simulink model "TCS_test_2"  (R2026a)
settings: Solver=ode4  StartTime=0  StopTime=5  FixedStep=0.0005
model workspace (MAT data in the model file):
  P.g = 9.81
  P.vehicleMass = 310
  P.channelMass = 155
  P.rearStaticFraction = 0.5
  P.wheelbase = 1.55
  P.cgHeight = 0.289
  P.tyreRadius = 0.25908
  P.gearRatio = 6
  P.drivetrainEfficiency = 0.95
  P.differentialSplit = 0.5
  P.motorPeakTorque = 220
  P.motorPeakPower = 80000
  P.motorMaximumRPM = 5170
  P.motorTimeConstant = 0.02
  P.wheelEquivalentInertia = 0.9
  P.rollingResistance = 0.015
  P.airDensity = 1.225
  P.dragArea = 0.8
  P.magicB = 10
  P.magicC = 1.9
  P.magicE = 0.97
  P.actualMuDry = 1.2
  P.actualMuLow = 0.48
  P.estimatedMuDry = 1.05
  P.estimatedMuLow = 0.58
  P.gripChangeTime = 1.5
  P.controllerSampleTime = 0.002
  P.plantStep = 0.0005
  P.stopTime = 5
  P.slipDenominatorGuard = 0.5
  P.slipFilterTimeConstant = 0.015
  P.slipTarget = 0.12
  P.slipActivation = 0.14
  P.slipRelease = 0.09
  P.activationPersistence = 0.02
  P.releasePersistence = 0.08
  P.recoveryTime = 0.12
  P.controlEnableSpeed = 1.5
  P.launchSlipVelocity = 0.35
  P.launchVelocityGain = 80
  P.launchTorqueCap = 85
  P.admissibleTorqueSafetyFactor = 0.95
  P.Kp = 650
  P.Ki = 900
  P.Kaw = 0.00153846153846
  P.integratorMinimum = -0.35
  P.integratorMaximum = 0.1
  P.torqueCutRate = 9000
  P.torqueRestoreRate = 500
  P.sensorResolutionRPM = 0.25
  P.faultTorque = 0
  driverProfile = [0  0; 0.2  0; 0.8  1; 2.8  1; 3  0; 3.3  0; 3.5  -0.8; 5.5  -0.8; 6  0]
  roadProfile = [0  1.2; 1.5  0.7; 2  1.2; 4  0.7; 4.5  1.2; 6  1.2]
libraries: simulink x1
Description:
  | Interactive single-wheel EV traction-control model.
  | Generated by build_TCS_test_2_simulink.m.
  | Proactive admissible torque plus reactive slip control.
settings Model: Creator=Arulm  LastModifiedBy=Arulm
settings DebuggingCC: AlgebraicLoopMsg=error  UnconnectedInputMsg=error  UnconnectedOutputMsg=error

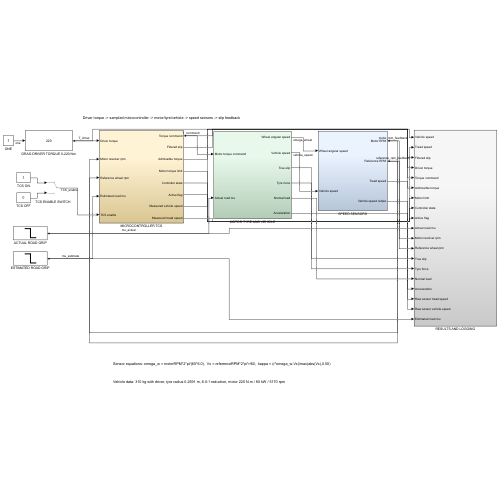
[thumbnail: Simulink's stored preview of the top-level diagram]
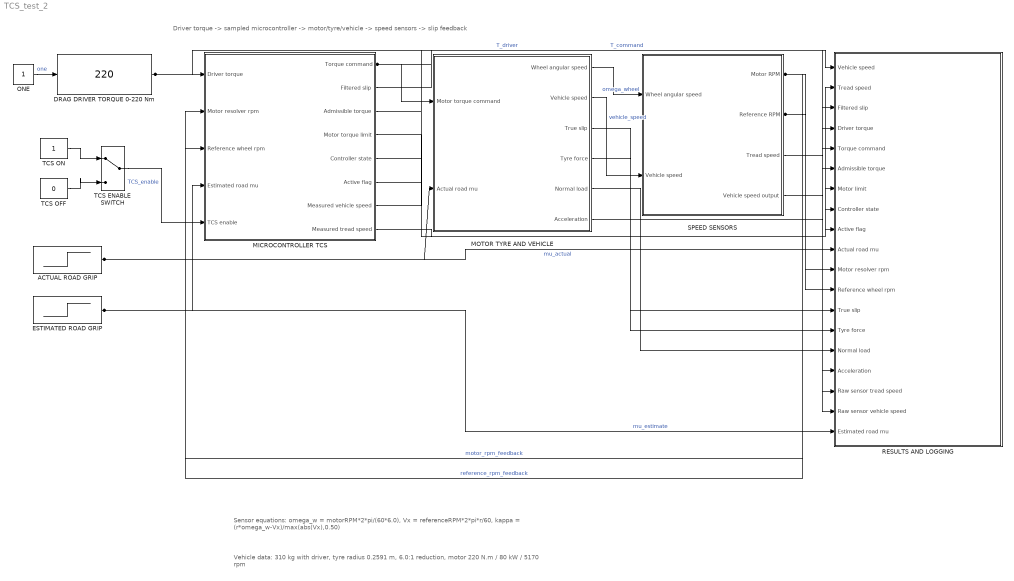
== system TCS_test_2 ==
  note: Driver torque -> sampled microcontroller -> motor/tyre/vehicle -> speed sensors -> slip feedback
  note: Sensor equations: omega_w = motorRPM*2*pi/(60*6.0), Vx = referenceRPM*2*pi*r/60, kappa = (r*omega_w-Vx)/max(abs(Vx),0.50)
  note: Vehicle data: 310 kg with driver, tyre radius 0.2591 m, 6.0:1 reduction, motor 220 N.m / 80 kW / 5170 rpm
  ACTUAL ROAD GRIP : Step  Time=1.5  InitialValue=1.2  FinalValue=0.48  SampleTime=0
  DRAG DRIVER TORQUE 0-220 Nm : simulink/Math Operations/Slider Gain  gain=220  low=0  high=220
  ESTIMATED ROAD GRIP : Step  Time=1.5  InitialValue=1.05  FinalValue=0.58  SampleTime=0
  MICROCONTROLLER TCS : Subsystem
  MOTOR TYRE AND VEHICLE : Subsystem
  ONE : Constant
  RESULTS AND LOGGING : Subsystem
  SPEED SENSORS : Subsystem
  TCS ENABLE SWITCH : ManualSwitch
  TCS OFF : Constant  Value=0  OutDataTypeStr=boolean
  TCS ON : Constant  OutDataTypeStr=boolean
  wires:
  ONE/1 -> DRAG DRIVER TORQUE 0-220 Nm/1  "one"
  TCS ON/1 -> TCS ENABLE SWITCH/1
  TCS OFF/1 -> TCS ENABLE SWITCH/2
  DRAG DRIVER TORQUE 0-220 Nm/1 -> MICROCONTROLLER TCS/1(Driver torque), RESULTS AND LOGGING/4(Driver torque)  "T_driver"
  TCS ENABLE SWITCH/1 -> MICROCONTROLLER TCS/5(TCS enable)  "TCS_enable"
  ESTIMATED ROAD GRIP/1 -> MICROCONTROLLER TCS/4(Estimated road mu), RESULTS AND LOGGING/19(Estimated road mu)  "mu_estimate"
  MICROCONTROLLER TCS/1(Torque command) -> MOTOR TYRE AND VEHICLE/1(Motor torque command), RESULTS AND LOGGING/5(Torque command)  "T_command"
  ACTUAL ROAD GRIP/1 -> MOTOR TYRE AND VEHICLE/2(Actual road mu), RESULTS AND LOGGING/10(Actual road mu)  "mu_actual"
  MOTOR TYRE AND VEHICLE/1(Wheel angular speed) -> SPEED SENSORS/1(Wheel angular speed)  "omega_wheel"
  MOTOR TYRE AND VEHICLE/2(Vehicle speed) -> SPEED SENSORS/2(Vehicle speed)  "vehicle_speed"
  SPEED SENSORS/1(Motor RPM) -> MICROCONTROLLER TCS/2(Motor resolver rpm), RESULTS AND LOGGING/11(Motor resolver rpm)  "motor_rpm_feedback"
  SPEED SENSORS/2(Reference RPM) -> MICROCONTROLLER TCS/3(Reference wheel rpm), RESULTS AND LOGGING/12(Reference wheel rpm)  "reference_rpm_feedback"
  MICROCONTROLLER TCS/7(Measured vehicle speed) -> RESULTS AND LOGGING/1(Vehicle speed)
  MICROCONTROLLER TCS/8(Measured tread speed) -> RESULTS AND LOGGING/2(Tread speed)
  MICROCONTROLLER TCS/2(Filtered slip) -> RESULTS AND LOGGING/3(Filtered slip)
  MICROCONTROLLER TCS/3(Admissible torque) -> RESULTS AND LOGGING/6(Admissible torque)
  MICROCONTROLLER TCS/4(Motor torque limit) -> RESULTS AND LOGGING/7(Motor limit)
  MICROCONTROLLER TCS/5(Controller state) -> RESULTS AND LOGGING/8(Controller state)
  MICROCONTROLLER TCS/6(Active flag) -> RESULTS AND LOGGING/9(Active flag)
  MOTOR TYRE AND VEHICLE/3(True slip) -> RESULTS AND LOGGING/13(True slip)
  MOTOR TYRE AND VEHICLE/4(Tyre force) -> RESULTS AND LOGGING/14(Tyre force)
  MOTOR TYRE AND VEHICLE/5(Normal load) -> RESULTS AND LOGGING/15(Normal load)
  MOTOR TYRE AND VEHICLE/6(Acceleration) -> RESULTS AND LOGGING/16(Acceleration)
  SPEED SENSORS/3(Tread speed) -> RESULTS AND LOGGING/17(Raw sensor tread speed)
  SPEED SENSORS/4(Vehicle speed output) -> RESULTS AND LOGGING/18(Raw sensor vehicle speed)

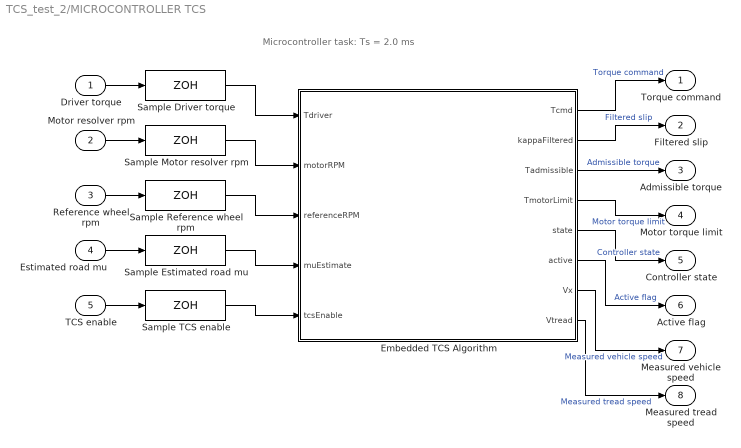
== system TCS_test_2/MICROCONTROLLER TCS ==
  note: Microcontroller task: Ts = 2.0 ms
  Driver torque : Inport
  Motor resolver rpm : Inport  Port=2
  Reference wheel rpm : Inport  Port=3
  Estimated road mu : Inport  Port=4
  TCS enable : Inport  Port=5
  Embedded TCS Algorithm : MATLAB Function  TreatAsAtomicUnit=on
  Sample Driver torque : ZeroOrderHold  SampleTime=0.002
  Sample Estimated road mu : ZeroOrderHold  SampleTime=0.002
  Sample Motor resolver rpm : ZeroOrderHold  SampleTime=0.002
  Sample Reference wheel rpm : ZeroOrderHold  SampleTime=0.002
  Sample TCS enable : ZeroOrderHold  SampleTime=0.002
  Torque command : Outport
  Filtered slip : Outport  Port=2
  Admissible torque : Outport  Port=3
  Motor torque limit : Outport  Port=4
  Controller state : Outport  Port=5
  Active flag : Outport  Port=6
  Measured vehicle speed : Outport  Port=7
  Measured tread speed : Outport  Port=8
  wires:
  Driver torque/1 -> Sample Driver torque/1
  Sample Driver torque/1 -> Embedded TCS Algorithm/1(Tdriver)
  Motor resolver rpm/1 -> Sample Motor resolver rpm/1
  Sample Motor resolver rpm/1 -> Embedded TCS Algorithm/2(motorRPM)
  Reference wheel rpm/1 -> Sample Reference wheel rpm/1
  Sample Reference wheel rpm/1 -> Embedded TCS Algorithm/3(referenceRPM)
  Estimated road mu/1 -> Sample Estimated road mu/1
  Sample Estimated road mu/1 -> Embedded TCS Algorithm/4(muEstimate)
  TCS enable/1 -> Sample TCS enable/1
  Sample TCS enable/1 -> Embedded TCS Algorithm/5(tcsEnable)
  Embedded TCS Algorithm/1(Tcmd) -> Torque command/1  "Torque command"
  Embedded TCS Algorithm/2(kappaFiltered) -> Filtered slip/1  "Filtered slip"
  Embedded TCS Algorithm/3(Tadmissible) -> Admissible torque/1  "Admissible torque"
  Embedded TCS Algorithm/4(TmotorLimit) -> Motor torque limit/1  "Motor torque limit"
  Embedded TCS Algorithm/5(state) -> Controller state/1  "Controller state"
  Embedded TCS Algorithm/6(active) -> Active flag/1  "Active flag"
  Embedded TCS Algorithm/7(Vx) -> Measured vehicle speed/1  "Measured vehicle speed"
  Embedded TCS Algorithm/8(Vtread) -> Measured tread speed/1  "Measured tread speed"

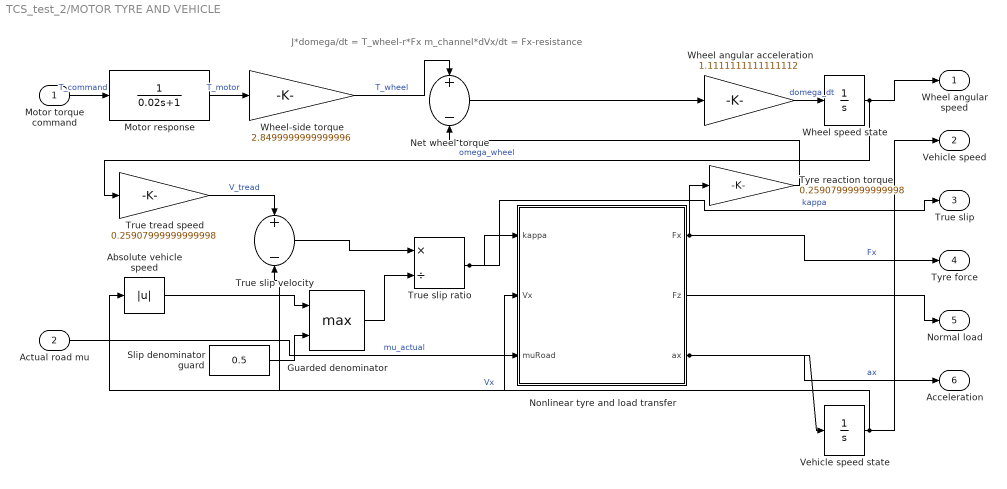
== system TCS_test_2/MOTOR TYRE AND VEHICLE ==
  note: J*domega/dt = T_wheel-r*Fx m_channel*dVx/dt = Fx-resistance
  Motor torque command : Inport
  Actual road mu : Inport  Port=2
  Absolute vehicle speed : Abs  SaturateOnIntegerOverflow=off
  Guarded denominator : MinMax  Function=max  Inputs=2
  Motor response : TransferFcn  Numerator=1  Denominator=[0.02 1]
  Net wheel torque : Sum  Inputs=+-
  Nonlinear tyre and load transfer : MATLAB Function  TreatAsAtomicUnit=on
  Slip denominator guard : Constant  Value=0.5
  True slip ratio : Product  Inputs=*/
  True slip velocity : Sum  Inputs=+-
  True tread speed : Gain  Gain=0.25907999999999998
  Tyre reaction torque : Gain  Gain=0.25907999999999998
  Vehicle speed state : Integrator  LimitOutput=on  LowerSaturationLimit=0
  Wheel angular acceleration : Gain  Gain=1.1111111111111112
  Wheel speed state : Integrator  LimitOutput=on  LowerSaturationLimit=0
  Wheel-side torque : Gain  Gain=2.8499999999999996
  Wheel angular speed : Outport
  Vehicle speed : Outport  Port=2
  True slip : Outport  Port=3
  Tyre force : Outport  Port=4
  Normal load : Outport  Port=5
  Acceleration : Outport  Port=6
  wires:
  Motor torque command/1 -> Motor response/1  "T_command"
  Motor response/1 -> Wheel-side torque/1  "T_motor"
  Wheel-side torque/1 -> Net wheel torque/1  "T_wheel"
  Wheel speed state/1 -> True tread speed/1, Wheel angular speed/1  "omega_wheel"
  True tread speed/1 -> True slip velocity/1  "V_tread"
  Vehicle speed state/1 -> True slip velocity/2, Absolute vehicle speed/1, Nonlinear tyre and load transfer/2(Vx), Vehicle speed/1  "Vx"
  Absolute vehicle speed/1 -> Guarded denominator/1
  Slip denominator guard/1 -> Guarded denominator/2
  True slip velocity/1 -> True slip ratio/1
  Guarded denominator/1 -> True slip ratio/2
  True slip ratio/1 -> Nonlinear tyre and load transfer/1(kappa), True slip/1  "kappa"
  Actual road mu/1 -> Nonlinear tyre and load transfer/3(muRoad)  "mu_actual"
  Nonlinear tyre and load transfer/1(Fx) -> Tyre reaction torque/1, Tyre force/1  "Fx"
  Tyre reaction torque/1 -> Net wheel torque/2
  Net wheel torque/1 -> Wheel angular acceleration/1
  Wheel angular acceleration/1 -> Wheel speed state/1  "domega_dt"
  Nonlinear tyre and load transfer/3(ax) -> Vehicle speed state/1, Acceleration/1  "ax"
  Nonlinear tyre and load transfer/2(Fz) -> Normal load/1

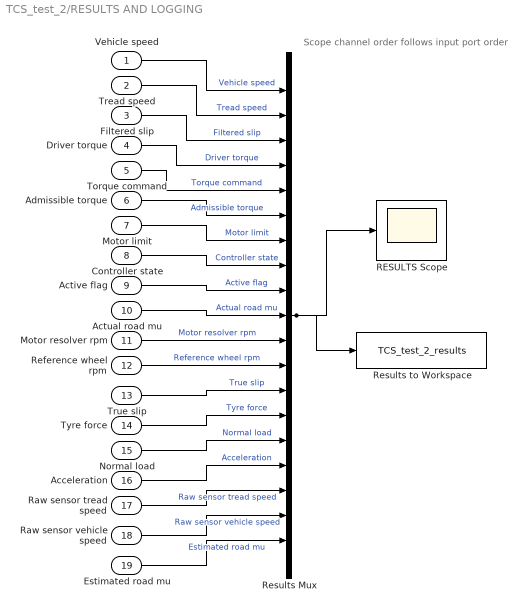
== system TCS_test_2/RESULTS AND LOGGING ==
  note: Scope channel order follows input port order
  Vehicle speed : Inport
  Tread speed : Inport  Port=2
  Filtered slip : Inport  Port=3
  Driver torque : Inport  Port=4
  Torque command : Inport  Port=5
  Admissible torque : Inport  Port=6
  Motor limit : Inport  Port=7
  Controller state : Inport  Port=8
  Active flag : Inport  Port=9
  Actual road mu : Inport  Port=10
  Motor resolver rpm : Inport  Port=11
  Reference wheel rpm : Inport  Port=12
  True slip : Inport  Port=13
  Tyre force : Inport  Port=14
  Normal load : Inport  Port=15
  Acceleration : Inport  Port=16
  Raw sensor tread speed : Inport  Port=17
  Raw sensor vehicle speed : Inport  Port=18
  Estimated road mu : Inport  Port=19
  RESULTS Scope : Scope
  Results Mux : Mux  Inputs=19
  Results to Workspace : ToWorkspace  VariableName=TCS_test_2_results  SaveFormat=Structure With Time  SampleTime=-1
  wires:
  Vehicle speed/1 -> Results Mux/1  "Vehicle speed"
  Tread speed/1 -> Results Mux/2  "Tread speed"
  Filtered slip/1 -> Results Mux/3  "Filtered slip"
  Driver torque/1 -> Results Mux/4  "Driver torque"
  Torque command/1 -> Results Mux/5  "Torque command"
  Admissible torque/1 -> Results Mux/6  "Admissible torque"
  Motor limit/1 -> Results Mux/7  "Motor limit"
  Controller state/1 -> Results Mux/8  "Controller state"
  Active flag/1 -> Results Mux/9  "Active flag"
  Actual road mu/1 -> Results Mux/10  "Actual road mu"
  Motor resolver rpm/1 -> Results Mux/11  "Motor resolver rpm"
  Reference wheel rpm/1 -> Results Mux/12  "Reference wheel rpm"
  True slip/1 -> Results Mux/13  "True slip"
  Tyre force/1 -> Results Mux/14  "Tyre force"
  Normal load/1 -> Results Mux/15  "Normal load"
  Acceleration/1 -> Results Mux/16  "Acceleration"
  Raw sensor tread speed/1 -> Results Mux/17  "Raw sensor tread speed"
  Raw sensor vehicle speed/1 -> Results Mux/18  "Raw sensor vehicle speed"
  Estimated road mu/1 -> Results Mux/19  "Estimated road mu"
  Results Mux/1 -> RESULTS Scope/1, Results to Workspace/1

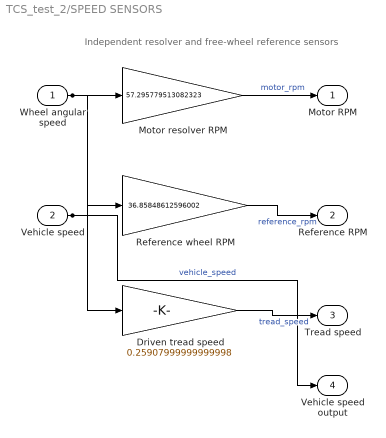
== system TCS_test_2/SPEED SENSORS ==
  note: Independent resolver and free-wheel reference sensors
  Wheel angular speed : Inport
  Vehicle speed : Inport  Port=2
  Driven tread speed : Gain  Gain=0.25907999999999998
  Motor resolver RPM : Gain  Gain=57.295779513082323
  Reference wheel RPM : Gain  Gain=36.85848612596002
  Motor RPM : Outport
  Reference RPM : Outport  Port=2
  Tread speed : Outport  Port=3
  Vehicle speed output : Outport  Port=4
  wires:
  Wheel angular speed/1 -> Motor resolver RPM/1, Driven tread speed/1
  Vehicle speed/1 -> Reference wheel RPM/1, Vehicle speed output/1  "vehicle_speed"
  Motor resolver RPM/1 -> Motor RPM/1  "motor_rpm"
  Reference wheel RPM/1 -> Reference RPM/1  "reference_rpm"
  Driven tread speed/1 -> Tread speed/1  "tread_speed"

== matlab function TCS_test_2/MOTOR TYRE AND VEHICLE/Nonlinear tyre and load transfer ==
  data: kappa input; Fx output; Vx input; muRoad input; Fz output; ax output
function [Fx,Fz,ax] = tyreVehicle(kappa,Vx,muRoad)
%#codegen
m = 310;
g = 9.8100000000000005;
rearFraction = 0.5;
h = 0.28899999999999998;
L = 1.55;
Crr = 0.014999999999999999;
rho = 1.2250000000000001;
CdA = 0.80000000000000004;
B = 10;
C = 1.8999999999999999;
E = 0.96999999999999997;
k = min(max(kappa,-5.0),5.0);
argument = B*k-E*(B*k-atan(B*k));
shape = sin(C*atan(argument));
q = max(muRoad,0.0)*shape;
rollingForce = Crr*m*g*tanh(Vx/0.20);
dragForce = 0.5*rho*CdA*Vx*abs(Vx);
resistancePerMass = (rollingForce+dragForce)/m;
denominator = max(1.0-q*h/L,0.25);
ax = (q*g*rearFraction-resistancePerMass)/denominator;
Fz = max((m*g*rearFraction+m*ax*h/L)/2.0,0.0);
Fx = q*Fz;
end

== matlab function TCS_test_2/MICROCONTROLLER TCS/Embedded TCS Algorithm ==
  settings: updateMethod=DISCRETE  sampleTime=0.002
  data: Tdriver input; Tcmd output; motorRPM input; referenceRPM input; muEstimate input; tcsEnable input; kappaFiltered output; Tadmissible output; TmotorLimit output; state output; active output; Vx output; Vtread output
function [Tcmd,kappaFiltered,Tadmissible,TmotorLimit,state,active,Vx,Vtread] = tcsController(Tdriver,motorRPM,referenceRPM,muEstimate,tcsEnable)
%#codegen
% Sampled single-wheel traction controller.
persistent kFilter z previousCommand stateMemory activationTimer releaseTimer recoveryTimer previousVx accelerationFilter
if isempty(kFilter)
    kFilter = 0.0; z = 0.0; previousCommand = 0.0;
    stateMemory = 0.0; activationTimer = 0.0; releaseTimer = 0.0;
    recoveryTimer = 0.0; previousVx = 0.0; accelerationFilter = 0.0;
end
Ts = 0.002;
r = 0.25907999999999998;
G = 6;
eta = 0.94999999999999996;
diffSplit = 0.5;
mass = 310;
g = 9.8100000000000005;
rearFraction = 0.5;
h = 0.28899999999999998;
L = 1.55;
Tpeak = 220;
Ppeak = 80000;
rpmMaximum = 5170;
rpmResolution = 0.25;
vGuard = 0.5;
tauFilter = 0.014999999999999999;
kappaTarget = 0.12;
kappaOn = 0.14000000000000001;
kappaOff = 0.089999999999999997;
enableSpeed = 1.5;
activationTime = 0.02;
releaseTime = 0.080000000000000002;
recoveryTimeLimit = 0.12;
launchSlipVelocity = 0.34999999999999998;
launchVelocityGain = 80;
launchTorque = 85;
safetyFactor = 0.94999999999999996;
Kp = 650;
Ki = 900;
Kaw = 0.0015384615384615385;
zMinimum = -0.34999999999999998;
zMaximum = 0.10000000000000001;
cutRate = 9000;
restoreRate = 500;
faultTorque = 0;

% Quantised sensor measurements.
motorRPMq = rpmResolution*round(motorRPM/rpmResolution);
referenceRPMq = rpmResolution*round(referenceRPM/rpmResolution);
sensorValid = isfinite(motorRPMq) && isfinite(referenceRPMq) && motorRPMq >= 0.0 && referenceRPMq >= 0.0;
if sensorValid
    omegaWheel = motorRPMq*(2.0*pi/60.0)/G;
    Vtread = r*omegaWheel;
    Vx = referenceRPMq*(2.0*pi/60.0)*r;
    slipVelocity = Vtread-Vx;
    kappaRaw = slipVelocity/max(abs(Vx),vGuard);
    kappaRaw = min(max(kappaRaw,-3.0),3.0);
else
    Vx = previousVx; Vtread = Vx; slipVelocity = 0.0; kappaRaw = 0.0;
end
alpha = Ts/(tauFilter+Ts);
kFilter = kFilter+alpha*(kappaRaw-kFilter);
kappaFiltered = kFilter;

% Physical motor torque-speed envelope.
omegaMotor = max(abs(motorRPMq)*2.0*pi/60.0,1.0);
if ~sensorValid || motorRPMq >= rpmMaximum
    TmotorLimit = 0.0;
else
    TmotorLimit = min(Tpeak,Ppeak/omegaMotor);
end

% Longitudinal load estimate for precautionary torque.
rawAcceleration = min(max((Vx-previousVx)/Ts,-15.0),15.0);
accelerationFilter = accelerationFilter+0.15*(rawAcceleration-accelerationFilter);
previousVx = Vx;
rearLoad = mass*g*rearFraction+mass*accelerationFilter*h/L;
FzEstimate = max(rearLoad/2.0,0.0);
Tadmissible = safetyFactor*max(muEstimate,0.0)*FzEstimate*r/(G*eta*diffSplit);
Tadmissible = min(max(Tadmissible,0.0),TmotorLimit);

requested = min(max(Tdriver,0.0),TmotorLimit);
lowSpeed = Vx < enableSpeed;
if lowSpeed
    launchFeedback = max(launchTorque-launchVelocityGain*max(slipVelocity-launchSlipVelocity,0.0),0.0);
    proactiveCap = min(requested,min(Tadmissible,launchFeedback));
else
    proactiveCap = min(requested,Tadmissible);
end

% State supervisor: 0 OFF, 1 LAUNCH, 2 ARMED, 3 ACTIVE, 4 RECOVERY, 5 FAULT.
if ~sensorValid
    stateMemory = 5.0;
elseif tcsEnable == 0 || requested < 0.01
    stateMemory = 0.0;
    activationTimer = 0.0; releaseTimer = 0.0; recoveryTimer = 0.0;
elseif lowSpeed
    stateMemory = 1.0;
    activationTimer = 0.0; releaseTimer = 0.0; recoveryTimer = 0.0;
else
    if stateMemory == 0.0 || stateMemory == 1.0 || stateMemory == 5.0
        stateMemory = 2.0;
    end
    if kFilter > kappaOn
        activationTimer = activationTimer+Ts;
    else
        activationTimer = 0.0;
    end
    if kFilter < kappaOff
        releaseTimer = releaseTimer+Ts;
    else
        releaseTimer = 0.0;
    end
    if stateMemory == 2.0 && activationTimer >= activationTime
        stateMemory = 3.0; releaseTimer = 0.0;
    elseif stateMemory == 3.0 && releaseTimer >= releaseTime
        stateMemory = 4.0; recoveryTimer = 0.0;
    elseif stateMemory == 4.0
        if kFilter > kappaOn
            stateMemory = 3.0; releaseTimer = 0.0;
        else
            recoveryTimer = recoveryTimer+Ts;
            if recoveryTimer >= recoveryTimeLimit
                stateMemory = 2.0; recoveryTimer = 0.0;
            end
        end
    end
end

if stateMemory == 3.0
    active = 1.0;
else
    active = 0.0;
end
if active ~= 0.0
    slipError = kappaTarget-kFilter;
    unsaturatedCap = proactiveCap+Kp*slipError+Ki*z;
    reactiveCap = min(max(unsaturatedCap,0.0),proactiveCap);
    zDerivative = slipError+Kaw*(reactiveCap-unsaturatedCap);
    z = min(max(z+Ts*zDerivative,zMinimum),zMaximum);
else
    reactiveCap = proactiveCap;
    if stateMemory ~= 4.0
        z = 0.0;
    end
end

if stateMemory == 5.0
    desiredTorque = faultTorque;
elseif tcsEnable ~= 0
    desiredTorque = reactiveCap;
else
    desiredTorque = requested;
end
if stateMemory == 5.0
    Tcmd = faultTorque;
else
    torqueChange = desiredTorque-previousCommand;
    torqueChange = min(max(torqueChange,-cutRate*Ts),restoreRate*Ts);
    Tcmd = min(max(previousCommand+torqueChange,0.0),TmotorLimit);
end
previousCommand = Tcmd;
state = stateMemory;
end
